simulink model "flyback"  (R2022b)
settings: Solver=VariableStepAuto  StartTime=0.0  StopTime=1  RelTol=1e-3
libraries: spsCurrentMeasurementLib x3, spsSeriesRLCBranchLib x3, spsDCVoltageSourceLib x1, spsDiodeLib x1, spsLinearTransformerLib x1, spsMosfetLib x1, simulink x1, spsVariableRatioTransformerLib x1, spsVoltageMeasurementLib x1, sps_lib x1
settings Model: Creator=Mehmet Emre Doğan  LastModifiedBy=Mehmet Emre Doğan

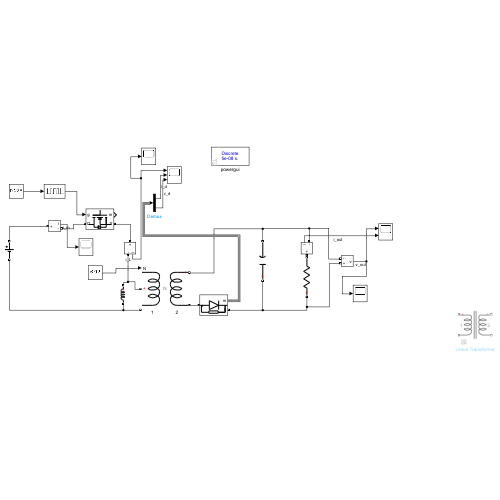
[thumbnail: Simulink's stored preview of the top-level diagram]
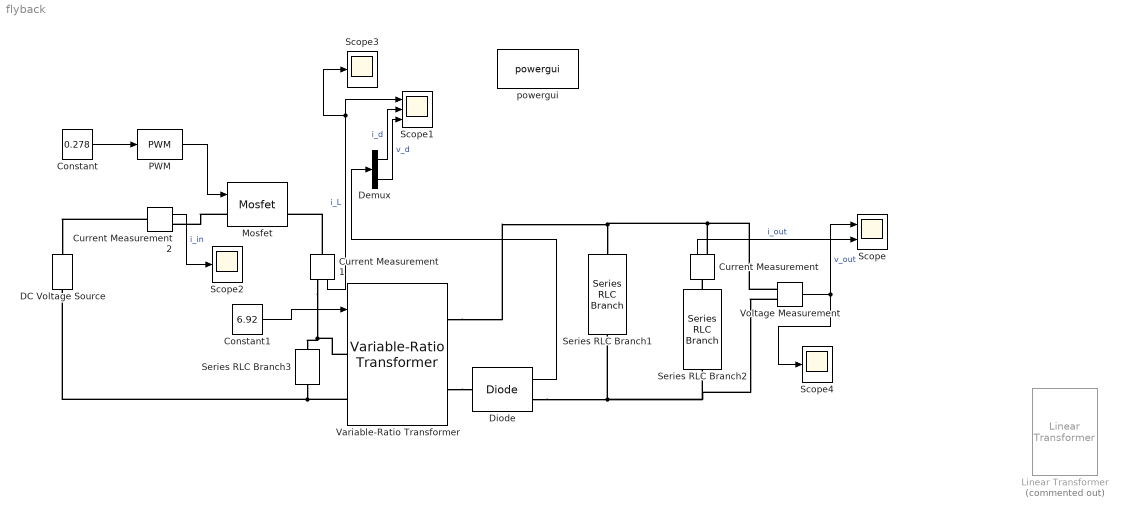
== system flyback ==
  Constant : Constant  Value=0.278
  Constant1 : Constant  Value=6.92
  Current Measurement : spsCurrentMeasurementLib/Current Measurement  PhasorSimulation=off  OutputType=Complex  PSBequivalent=0
  Current Measurement1 : spsCurrentMeasurementLib/Current Measurement  PhasorSimulation=off  OutputType=Complex  PSBequivalent=0
  Current Measurement2 : spsCurrentMeasurementLib/Current Measurement  PhasorSimulation=off  OutputType=Complex  PSBequivalent=0
  DC Voltage Source : spsDCVoltageSourceLib/DC Voltage Source  Amplitude=18  Measurements=None
  Demux : Demux  Outputs=2
  Diode : spsDiodeLib/Diode  Ron=0.001  Lon=0  Vf=0.8e-3  IC=0  UseSnubber=0  Rs=500e3  Cs=250e-9  Measurements=on
  Linear Transformer : spsLinearTransformerLib/Linear Transformer  Commented=on  UNITS=SI  NominalPower=[100 100e3]  winding1=[12 10.48e-3 56e-9]  winding2=[48 252.6e-3 56e-9]  ThreeWindings=off  winding3=[3.15e+05 0.7938 0.084225]  RmLm=[6.75, 8e-6]  Measurements=None  DataType=on
  Mosfet : spsMosfetLib/Mosfet  Ron=0.1e-3  Lon=0  Rd=0.01e-3  Vfd=0  IC=0  Rs=1e5  Cs=inf  Measurements=on
  PWM : simulink/Discontinuities/PWM  DisableCoverage=on  Period=1/(100e3)  InitialDelay=0  DisallowZeroDutyCycle=on  RunAtFixedTimeIntervals=off  SampleTime=0.1
  Scope : Scope  NumInputPorts=2
  Scope1 : Scope  NumInputPorts=3
  Scope2 : Scope
  Scope3 : Scope
  Scope4 : Scope
  Series RLC Branch1 : spsSeriesRLCBranchLib/Series RLC Branch  LConnTagsString=__new0  RConnTagsString=__new0  BranchType=C  Resistance=1  Inductance=1e-3  SetiL0=off  InitialCurrent=0  Capacitance=52e-6  Setx0=off  InitialVoltage=0  Measurements=None
  Series RLC Branch2 : spsSeriesRLCBranchLib/Series RLC Branch  LConnTagsString=__new0  RConnTagsString=__new0  BranchType=R  Resistance=48  Inductance=1e-3  SetiL0=off  InitialCurrent=0  Capacitance=1e-6  Setx0=off  InitialVoltage=0  Measurements=None
  Series RLC Branch3 : spsSeriesRLCBranchLib/Series RLC Branch  LConnTagsString=__new0  RConnTagsString=__new0  BranchType=L  Resistance=1  Inductance=8e-6  SetiL0=off  InitialCurrent=0  Capacitance=52e-6  Setx0=off  InitialVoltage=0  Measurements=None
  Variable-Ratio Transformer : spsVariableRatioTransformerLib/Variable-Ratio Transformer
      settings: LibrarySourceBlock=|
      | sps_lib/Passives/Variable-Ratio
      | Transformer
  Voltage Measurement : spsVoltageMeasurementLib/Voltage Measurement  PhasorSimulation=off  OutputType=Complex  PSBequivalent=0
  powergui : sps_lib/powergui  Priority=1  SimulationMode=Discrete  SampleTime=50e-9  frequency=60  Iterations=50  frequencyindice=0  Pbase=100e6  ErrMax=1e-4  UnitsV=kV  UnitsW=MW  buscounter=0  FunctionMessages=off  echomessages=off  EnableUseOfTLC=off  CurrentSourceSwitches=off  DisableSnubberDevices=off  DisableRonSwitches=off  DisableVfSwitches=off  DisplayEquations=off  AutomaticDiscreteSolvers=off  SolverType=Tustin/Backward Euler (TBE)  Interpol=off  ExternalGateDelay=off  methode=off  Ts=100  x0status=blocks  SPID=on  SwTol=0  HookPort=off  NonlinearTolerance=1e-4  nMaxIteration=100  ContinueOnMaxIteration=off  RestoreLinks=warning  ResistiveCurrentMeasurement=off  Frange=[0:2:500]  Ylog=off  Xlog=on  ShowGrid=off  save=off  variable=ZData  structure=0  ZoomFFT=off  StartTime=0.0  cycles=1  DisplayStyle=1  fundamental=60  FreqAxis=off  MaxFrequency=1000  frequencyindicesteady=1  RmsSteady=1  display=off
  wires:
  Constant/1 -> PWM/1
  PWM/1 -> Mosfet/1
  Voltage Measurement/1 -> Scope/1, Scope4/1  "v_out"
  Current Measurement/1 -> Scope/2  "i_out"
  Current Measurement1/1 -> Scope3/1, Scope1/1  "i_L"
  Current Measurement2/1 -> Scope2/1  "i_in"
  Demux/1 -> Scope1/2  "i_d"
  Demux/2 -> Scope1/3  "v_d"
  Diode/1 -> Demux/1
  Constant1/1 -> Variable-Ratio Transformer/1
  connections:
  Mosfet/LConn1 -- Current Measurement2/RConn1
  Current Measurement1/LConn1 -- Mosfet/RConn1
  Series RLC Branch2/LConn1 -- Voltage Measurement/LConn1 -- Series RLC Branch1/LConn1 -- Diode/RConn1
  Current Measurement1/RConn1 -- Variable-Ratio Transformer/LConn1 -- Series RLC Branch3/LConn1
  Series RLC Branch2/RConn1 -- Current Measurement/LConn1
  Current Measurement2/LConn1 -- DC Voltage Source/RConn1
  Series RLC Branch3/RConn1 -- Variable-Ratio Transformer/LConn2 -- DC Voltage Source/LConn1
  Voltage Measurement/LConn2 -- Current Measurement/RConn1 -- Variable-Ratio Transformer/RConn1 -- Series RLC Branch1/RConn1
  Variable-Ratio Transformer/RConn2 -- Diode/LConn1
